simulink model "sampleModel1719"  (R2023a)
settings: Solver=VariableStepAuto  StartTime=0.0  StopTime=10.0  RelTol=1e-3
libraries: hdlsllib x6, simulink x1
settings Model: Creator=user1  LastModifiedBy=user1

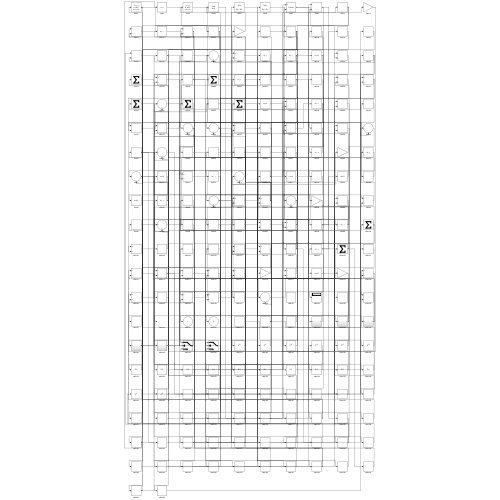
[thumbnail: Simulink's stored preview of the top-level diagram]
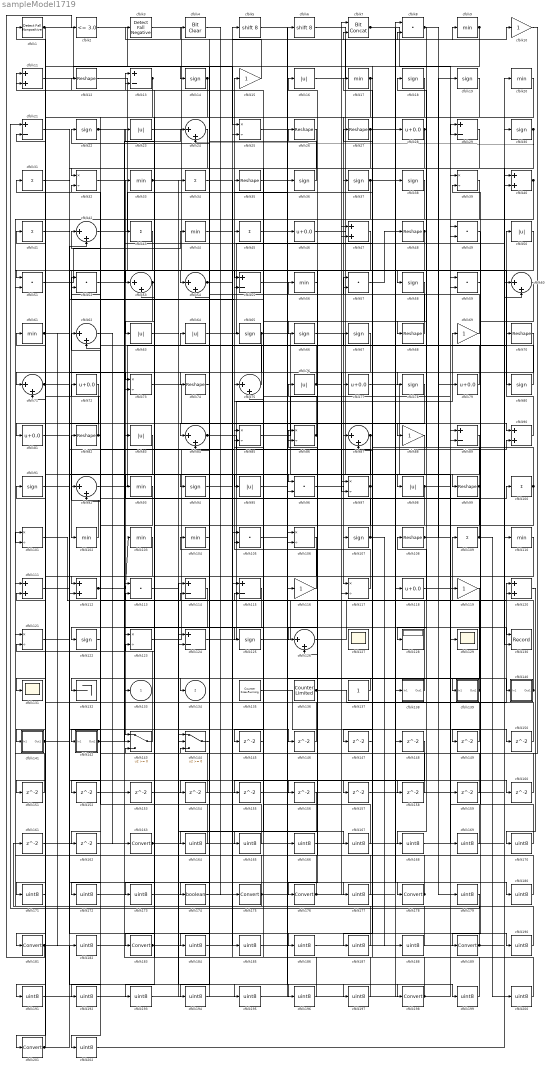
== system sampleModel1719 ==
  cfblk1 : hdlsllib/Logic and Bit Operations/Detect Fall Nonpositive  vinit=0  OutDataTypeStr=boolean
  cfblk{10,15,69,88,116,119} (6 alike) : Gain
  cfblk{31,34,41,43,45,100,109} (7 alike) : Sum  Inputs=+
  cfblk{25,32,39,73,85..86,97,101,106,117,121,123} (12 alike) : Product  Inputs=*/  RndMeth=Zero  SaturateOnIntegerOverflow=on
  cfblk{9,17,20,33,44,56,61,93,102..104,110} (12 alike) : MinMax
  cfblk{8,49,51..52,57,59,96,105,113} (9 alike) : DotProduct  OutDataTypeStr=Inherit: Inherit via internal rule
  cfblk{14,18..19,22,30,36..38,58,65..67,78,80,91,94,107,122,125} (19 alike) : Signum
  cfblk{12,26..27,35,48,68,70,74,82,99,108} (11 alike) : Reshape
  cfblk{11,40,47,90,111..112,120} (7 alike) : Sum
  cfblk{13,21,29,55,89,114..115,124} (8 alike) : Sum  Inputs=+-
  cfblk{28,46,72,77,79,81,118} (7 alike) : Bias  Bias=0.0  SaturateOnIntegerOverflow=off
  cfblk{24,42,53..54,60,62,71,75,84,87,92,126} (12 alike) : Sum  Inputs=|++
  cfblk127 : Scope
      settings: Floating=on
  cfblk128 : Display
  cfblk129 : Scope
  cfblk130 : Record  FileSettingsInternal="{\"entries\":[{\"content\":{\"excelSettings\":{\"content\":{},\"type\":\"Streamout.ExcelSettings\"}},\"type\":\"Streamout.FileSettingStorage\",\"uuid\":\"\"}],\"packageUris\":[\"http:\\/\\/schema.mathworks.com\\/mf0\\/streamout_blocks\\/R2020a\"],\"version\":\"1.0\"}"  Layout=[1 1]  SignalsInternal="{\"entries\":[{\"content\":{\"signals\":[{\"content\":{\"blockPath\":[],\"dimensions\":[1],\"domain\":\"\",\"lineColor\":\"#a2142f\",\"plots\":[1],\"port\":1,\"signalID\":3243,\"signalName\":\"XY Graph:1\"},\"type\":\"RecordBlkView.Signal\",\"uuid\":\"\"},{\"content\":{\"blockPath\":[],\"dimensions\":[1],\"domain\":\"\",\"lineColor\":\"#139fff\",\"plots\":[1],\"port\":2,\"signalID\":3246,\"signalName\":\"XY Graph:2\"},\"type\":\"RecordBlkView.Signal\",\"uuid\":\"\"}]},\"type\":\"RecordBlkView.InputSignals\",\"uuid\":\"\"}],\"packageUris\":[\"http:\\/\\/schema.mathworks.com\\/mf0\\/streamout_blocks\\/R2020a\"],\"version\":\"1.0\"}"  VisualizationBindings="{\"xyplotplugin\":{\"info\":[{\"series\":[{\"bindingParametersList\":[{\"parameter\":\"X-Axis\",\"signalID\":3243,\"signalName\":\"XY Graph:1\"},{\"parameter\":\"Y-Axis\",\"signalID\":3246,\"signalName\":\"XY Graph:2\"}],\"seriesID\":14732}],\"subplotID\":1}]}}"  CompatibilityTag=XY  st=-1
  cfblk131 : Scope
  cfblk132 : Terminator
  cfblk135 : hdlsllib/Sources/Counter Free-Running  NumBits=16  tsamp=-1
  cfblk136 : hdlsllib/Sources/Counter Limited  uplimit=7  tsamp=-1
  cfblk137 : Constant  SampleTime=-1
  cfblk138 : Subsystem
      settings: LibrarySourceBlock=|
      | hdlsllib/Ports &
      | Subsystems/Subsystem
  cfblk139 : Subsystem
      settings: LibrarySourceBlock=|
      | hdlsllib/Ports &
      | Subsystems/Subsystem
  cfblk140 : Subsystem
      settings: LibrarySourceBlock=|
      | hdlsllib/Ports &
      | Subsystems/Subsystem
  cfblk141 : Subsystem
      settings: LibrarySourceBlock=|
      | hdlsllib/Ports &
      | Subsystems/Subsystem
  cfblk142 : Subsystem
      settings: LibrarySourceBlock=|
      | hdlsllib/Ports &
      | Subsystems/Subsystem
  cfblk143 : Switch  SaturateOnIntegerOverflow=off  InputSameDT=off
  cfblk144 : Switch  SaturateOnIntegerOverflow=off  InputSameDT=off
  cfblk{145..162} (18 alike) : Delay  SampleTime=1
  cfblk{16,23,50,63..64,76,83,95,98} (9 alike) : Abs  SaturateOnIntegerOverflow=off
  cfblk{163,175..176,178,181,183,189,198,201} (9 alike) : DataTypeConversion  SaturateOnIntegerOverflow=off  RndMeth=Floor
  cfblk{164..173,177,179..180,182,184..188,190..197,199..200,202} (30 alike) : DataTypeConversion  OutDataTypeStr=uint8  SaturateOnIntegerOverflow=off  RndMeth=Floor
  cfblk174 : DataTypeConversion  OutDataTypeStr=boolean  SaturateOnIntegerOverflow=off  RndMeth=Floor
  cfblk2 : hdlsllib/Logic and Bit Operations/Compare To Constant  relop=<=  const=3.0  OutDataTypeStr=boolean
  cfblk3 : hdlsllib/Logic and Bit Operations/Detect Fall Negative  vinit=0  OutDataTypeStr=boolean
  cfblk4 : simulink/Logic and Bit Operations/Bit Clear  iBit=0
      settings: LibrarySourceBlock=|
      | hdlsllib/Logic and Bit
      | Operations/Bit Clear
  cfblk5 : ArithShift  BitShiftNumber=8
  cfblk6 : ArithShift  BitShiftNumber=8
  cfblk7 : hdlsllib/Logic and Bit Operations/Bit Concat  numInputs=2
  cfblk133 : Outport  VectorParamsAs1DForOutWhenUnconnected=off
  cfblk134 : Outport  Port=2  VectorParamsAs1DForOutWhenUnconnected=off
  wires:
  cfblk12/1 -> cfblk54/1
  cfblk116/1 -> cfblk15/1
  cfblk2/1 -> cfblk54/2
  cfblk43/1 -> cfblk102/1
  cfblk101/1 -> cfblk109/1
  cfblk17/1 -> cfblk117/1, cfblk123/1, cfblk96/2, cfblk187/1
  cfblk65/1 -> cfblk98/1, cfblk71/2
  cfblk102/1 -> cfblk82/1
  cfblk38/1 -> cfblk84/1
  cfblk61/1 -> cfblk73/2, cfblk160/1, cfblk182/1
  cfblk97/1 -> cfblk72/1, cfblk126/1, cfblk67/1
  cfblk90/1 -> cfblk50/1
  cfblk4/1 -> cfblk175/1
  cfblk26/1 -> cfblk75/2
  cfblk57/1 -> cfblk48/1
  cfblk93/1 -> cfblk142/1(In1)
  cfblk123/1 -> cfblk5/1
  cfblk107/1 -> cfblk33/1, cfblk32/2, cfblk188/1
  cfblk83/1 -> cfblk143/1
  cfblk3/1 -> cfblk80/1
  cfblk55/1 -> cfblk139/1(In1)
  cfblk124/1 -> cfblk69/1
  cfblk137/1 -> cfblk132/1
  cfblk82/1 -> cfblk122/1, cfblk41/1
  cfblk115/1 -> cfblk183/1
  cfblk117/1 -> cfblk16/1
  cfblk6/1 -> cfblk119/1
  cfblk8/1 -> cfblk128/1, cfblk179/1
  cfblk92/1 -> cfblk70/1
  cfblk16/1 -> cfblk9/1
  cfblk67/1 -> cfblk112/1
  cfblk11/1 -> cfblk14/1
  cfblk121/1 -> cfblk85/1
  cfblk77/1 -> cfblk129/1
  cfblk99/1 -> cfblk18/1, cfblk43/1, cfblk126/2
  cfblk19/1 -> cfblk51/1
  cfblk64/1 -> cfblk40/1
  cfblk41/1 -> cfblk53/1
  cfblk37/1 -> cfblk124/2, cfblk180/1
  cfblk96/1 -> cfblk107/1
  cfblk7/1 -> cfblk138/1(In1), cfblk29/2
  cfblk60/1 -> cfblk99/1
  cfblk20/1 -> cfblk201/1
  cfblk22/1 -> cfblk144/2, cfblk172/1
  cfblk112/1 -> cfblk103/1, cfblk153/1
  cfblk136/1 -> cfblk120/1, cfblk86/1
  cfblk71/1 -> cfblk90/1, cfblk88/1
  cfblk52/1 -> cfblk58/1
  cfblk138/1(Out1) -> cfblk23/1
  cfblk108/1 -> cfblk89/1, cfblk79/1
  cfblk72/1 -> cfblk81/1
  cfblk18/1 -> cfblk37/1
  cfblk139/1(Out1) -> cfblk92/1, cfblk104/1
  cfblk126/1 -> cfblk29/1
  cfblk141/1(Out1) -> cfblk120/2, cfblk55/2
  cfblk91/1 -> cfblk96/1
  cfblk110/1 -> cfblk181/1
  cfblk78/1 -> cfblk134/1
  cfblk23/1 -> cfblk60/2
  cfblk80/1 -> cfblk31/1
  cfblk14/1 -> cfblk73/1, cfblk191/1
  cfblk105/1 -> cfblk198/1
  cfblk51/1 -> cfblk44/1
  cfblk50/1 -> cfblk66/1
  cfblk28/1 -> cfblk68/1, cfblk55/1
  cfblk35/1 -> cfblk106/1
  cfblk46/1 -> cfblk118/1
  cfblk73/1 -> cfblk116/1
  cfblk40/1 -> cfblk51/2, cfblk164/1
  cfblk143/1 -> cfblk11/1
  cfblk53/1 -> cfblk143/2, cfblk93/1
  cfblk69/1 -> cfblk17/1
  cfblk66/1 -> cfblk77/1
  cfblk59/1 -> cfblk189/1
  cfblk32/1 -> cfblk130/1
  cfblk15/1 -> cfblk3/1
  cfblk125/1 -> cfblk8/1
  cfblk86/1 -> cfblk13/1, cfblk52/2, cfblk11/2
  cfblk87/1 -> cfblk131/1, cfblk57/1
  cfblk109/1 -> cfblk83/1, cfblk200/1
  cfblk21/1 -> cfblk178/1
  cfblk100/1 -> cfblk35/1, cfblk133/1, cfblk155/1
  cfblk10/1 -> cfblk143/3
  cfblk68/1 -> cfblk22/1
  cfblk5/1 -> cfblk106/2
  cfblk36/1 -> cfblk12/1
  cfblk56/1 -> cfblk176/1
  cfblk42/1 -> cfblk6/1
  cfblk33/1 -> cfblk34/1, cfblk190/1
  cfblk62/1 -> cfblk163/1
  cfblk70/1 -> cfblk97/2
  cfblk1/1 -> cfblk25/1, cfblk141/1(In1)
  cfblk140/1(Out1) -> cfblk26/1, cfblk108/1
  cfblk25/1 -> cfblk140/1(In1)
  cfblk84/1 -> cfblk90/2, cfblk7/2
  cfblk142/1(Out1) -> cfblk100/1, cfblk24/1
  cfblk9/1 -> cfblk87/1, cfblk71/1
  cfblk29/1 -> cfblk78/1
  cfblk79/1 -> cfblk52/1
  cfblk30/1 -> cfblk130/2, cfblk125/1, cfblk24/2
  cfblk75/1 -> cfblk64/1
  cfblk58/1 -> cfblk95/1
  cfblk98/1 -> cfblk19/1, cfblk147/1, cfblk150/1
  cfblk27/1 -> cfblk112/2, cfblk74/1, cfblk10/1
  cfblk13/1 -> cfblk92/2, cfblk32/1
  cfblk76/1 -> cfblk13/2, cfblk8/2
  cfblk48/1 -> cfblk101/2, cfblk63/1
  cfblk85/1 -> cfblk49/2
  cfblk54/1 -> cfblk94/1, cfblk156/1
  cfblk89/1 -> cfblk145/1
  cfblk145/1 -> cfblk75/1
  cfblk31/1 -> cfblk146/1
  cfblk146/1 -> cfblk1/1
  cfblk147/1 -> cfblk87/2
  cfblk49/1 -> cfblk149/1
  cfblk149/1 -> cfblk84/2
  cfblk150/1 -> cfblk57/2
  cfblk106/1 -> cfblk151/1
  cfblk151/1 -> cfblk101/1
  cfblk103/1 -> cfblk152/1
  cfblk152/1 -> cfblk117/2
  cfblk153/1 -> cfblk7/1
  cfblk74/1 -> cfblk154/1
  cfblk154/1 -> cfblk124/1
  cfblk94/1 -> cfblk157/1
  cfblk157/1 -> cfblk40/2
  cfblk81/1 -> cfblk158/1
  cfblk158/1 -> cfblk97/1
  cfblk118/1 -> cfblk159/1
  cfblk159/1 -> cfblk144/1
  cfblk160/1 -> cfblk42/1
  cfblk161/1 -> cfblk25/2
  cfblk122/1 -> cfblk162/1
  cfblk162/1 -> cfblk60/1
  cfblk163/1 -> cfblk38/1, cfblk89/2
  cfblk164/1 -> cfblk62/1
  cfblk148/1 -> cfblk165/1
  cfblk165/1 -> cfblk62/2
  cfblk45/1 -> cfblk166/1
  cfblk166/1 -> cfblk76/1
  cfblk63/1 -> cfblk167/1
  cfblk167/1 -> cfblk45/1
  cfblk39/1 -> cfblk168/1
  cfblk168/1 -> cfblk30/1
  cfblk135/1 -> cfblk169/1
  cfblk169/1 -> cfblk39/1
  cfblk120/1 -> cfblk170/1
  cfblk170/1 -> cfblk39/2
  cfblk47/1 -> cfblk171/1
  cfblk171/1 -> cfblk121/2
  cfblk172/1 -> cfblk47/1
  cfblk88/1 -> cfblk173/1
  cfblk173/1 -> cfblk47/2
  cfblk104/1 -> cfblk174/1
  cfblk174/1 -> cfblk4/1
  cfblk175/1 -> cfblk161/1, cfblk61/1
  cfblk176/1 -> cfblk148/1, cfblk85/2
  cfblk44/1 -> cfblk177/1
  cfblk177/1 -> cfblk56/1
  cfblk178/1 -> cfblk144/3, cfblk121/1
  cfblk179/1 -> cfblk21/1
  cfblk180/1 -> cfblk21/2
  cfblk181/1 -> cfblk2/1, cfblk196/1
  cfblk182/1 -> cfblk110/1
  cfblk183/1 -> cfblk86/2, cfblk36/1
  cfblk144/1 -> cfblk184/1
  cfblk184/1 -> cfblk115/1
  cfblk34/1 -> cfblk185/1
  cfblk185/1 -> cfblk115/2
  cfblk111/1 -> cfblk186/1
  cfblk186/1 -> cfblk49/1
  cfblk187/1 -> cfblk111/1
  cfblk188/1 -> cfblk111/2
  cfblk189/1 -> cfblk123/2, cfblk65/1
  cfblk190/1 -> cfblk59/1
  cfblk191/1 -> cfblk59/2
  cfblk114/1 -> cfblk192/1
  cfblk192/1 -> cfblk28/1
  cfblk119/1 -> cfblk193/1
  cfblk193/1 -> cfblk114/1
  cfblk156/1 -> cfblk194/1
  cfblk194/1 -> cfblk114/2
  cfblk113/1 -> cfblk195/1
  cfblk195/1 -> cfblk46/1
  cfblk196/1 -> cfblk113/1
  cfblk95/1 -> cfblk197/1
  cfblk197/1 -> cfblk113/2
  cfblk198/1 -> cfblk53/2, cfblk27/1
  cfblk155/1 -> cfblk199/1
  cfblk199/1 -> cfblk105/1
  cfblk200/1 -> cfblk105/2
  cfblk201/1 -> cfblk91/1, cfblk42/2
  cfblk24/1 -> cfblk202/1
  cfblk202/1 -> cfblk20/1

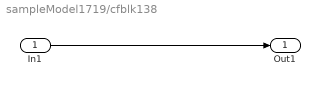
== system sampleModel1719/cfblk138 ==
  In1 : Inport
  Out1 : Outport
  wires:
  In1/1 -> Out1/1

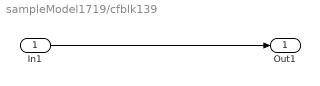
== system sampleModel1719/cfblk139 ==
  In1 : Inport
  Out1 : Outport
  wires:
  In1/1 -> Out1/1

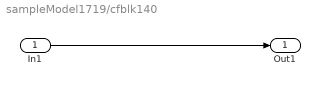
== system sampleModel1719/cfblk140 ==
  In1 : Inport
  Out1 : Outport
  wires:
  In1/1 -> Out1/1

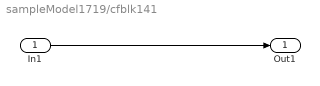
== system sampleModel1719/cfblk141 ==
  In1 : Inport
  Out1 : Outport
  wires:
  In1/1 -> Out1/1

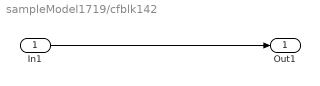
== system sampleModel1719/cfblk142 ==
  In1 : Inport
  Out1 : Outport
  wires:
  In1/1 -> Out1/1
